simulink model "traffic"  (R2020a)
settings: Solver=FixedStepDiscrete  StartTime=0.0  StopTime=12  FixedStep=0.01  RelTol=1e-3
settings Model: EnablePacing=on  Creator=avizinho  LastModifiedBy=avizinho

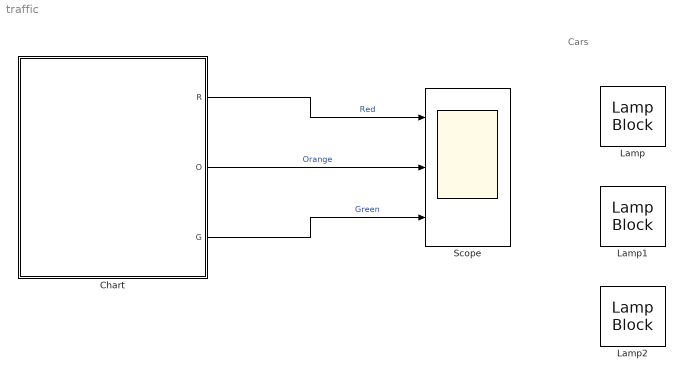
== system traffic ==
  note: Cars
  Chart : Stateflow chart  TreatAsAtomicUnit=on
  Lamp : LampBlock  LabelPosition=Hide
  Lamp1 : LampBlock  LabelPosition=Hide
  Lamp2 : LampBlock  LabelPosition=Hide
  Scope : Scope  NumInputPorts=3
  wires:
  Chart/1(R) -> Scope/1  "Red"
  Chart/2(O) -> Scope/2  "Orange"
  Chart/3(G) -> Scope/3  "Green"

== stateflow chart traffic/Chart ==
  state Red
    entry: R=1;
    exit: R=0;
  state Orange
    entry: O=1;
    exit: O=0;
  state Green
    entry: G=1;
    exit: G=0;
  (default) -> Red
  Red -> Green : after(2,sec)
  Orange -> Red : after(1,sec)
  Green -> Orange : after(3,sec)
  data: R output; O output; G output
